simulink model "Raspberry_Audio"  (R2020a)
settings: Solver=FixedStepDiscrete  StartTime=0.0  StopTime=inf  RelTol=1e-3  EnableMultiTasking=on
InitFcn:
  | audio_equalizer_data
  | audioSignal = audioread(fullfile(matlabroot,'toolbox','signal','signal','guitartune.wav'));
  | audioSignal = int16((2^15-1)*audioSignal);
StartFcn:
  | audio_equalizer_gui
undefined symbols (not defined in the file): CoeffsMatrix1, CoeffsMatrix2, CoeffsMatrix3, dfilt
libraries: dsparch4 x3, embdlinuxlib x1, dspsrcs4 x1
CloseFcn:
  | % Delete parameters
  | clear CoeffsMatrix1 CoeffsMatrix2  CoeffsMatrix3
  | clear coeffsMatrix1   coeffsMatrix2   coeffsMatrix3
  | clear in out
  | clear audiosamplingrate
  | 
  | % Delete GUI
  | delete(findall(0, 'type', 'figure', 'Name', 'Three Band Equalizer'));
  | 
  | % Clear audio signal
  | clear audioSignal
settings Model: SimulationMode=external  ExtModeTrigDuration=100  Creator=The MathWorks, Inc.  LastModifiedBy=miche
settings SolverCC: PositivePriorityOrder=on
settings DataIOCC: LimitDataPoints=on  SaveFormat=Array  ReturnWorkspaceOutputs=off
settings OptimizationCC: ExpressionDepthLimit=2147483647  LifeSpan=Inf  MaxStackSize=64
settings DebuggingCC: UnderspecifiedInitializationDetection=Classic  MergeDetectMultiDrivingBlocksExec=none  IntegerOverflowMsg=none  ParameterOverflowMsg=none  ParameterPrecisionLossMsg=none  FcnCallInpInsideContextMsg=warning  AllowSymbolicDim=off  StateNameClashWarn=warning  SFUnexpectedBacktrackingDiag=warning  SFNoUnconditionalDefaultTransitionDiag=warning  SFExecutionAtInitializationDiag=none  IntegerSaturationMsg=none  ArithmeticOperatorsInVariantConditions=warning
settings HardwareCC: ProdBitPerPointer=32  ProdBitPerSizeT=32  ProdBitPerPtrDiffT=32  ProdLargestAtomicInteger=Long  ProdLargestAtomicFloat=Double  ProdWordSize=32  ProdHWDeviceType=ARM Compatible->ARM Cortex  UseEmbeddedCoderFeatures=off  UseSimulinkCoderFeatures=off
settings ModelReferenceCC: PropagateSignalLabelsOutOfModel=off
settings SFSimCC: SimUseLocalCustomCode=off  CustomCodeUndefinedFunction=UseInterfaceOnly
settings RTWCC: SystemTargetFile=ert.tlc  HardwareBoard=Raspberry Pi  TLCOptions=-aInlineSetEventsForThisBaseRateFcn=TLC_FALSE -aSuppressMultiTaskScheduler=TLC_FALSE -aRateBasedStepFcn=0  TemplateMakefile=ert_default_tmf  GenerateReport=on  RTWVerbose=off  RTWUseLocalCustomCode=off  Toolchain=GNU GCC Raspberry Pi  LaunchReport=on
settings CodeAppCC: ForceParamTrailComments=on  OperatorAnnotations=on  StateflowObjectComments=on  MATLABSourceComments=on
settings ERTTargetCC: MultiwordLength=2048  ERTCustomFileBanners=off  SupportContinuousTime=on  SupportNonInlinedSFcns=on  RemoveResetFunc=off  ModelStepFunctionPrototypeControlCompliant=off
settings ConfigComp: CovMetricSettings=dw  CovHtmlReporting=on  CovSaveCumulativeToWorkspaceVar=on  CovSaveSingleToWorkspaceVar=on  CovShowResultsExplorer=off  CovExternalEMLEnable=off

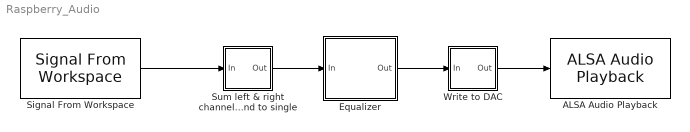
== system Raspberry_Audio ==
  ALSA Audio Playback : embdlinuxlib/ALSA Audio Playback  deviceStr='default'  sampleRateEnum=44100  queueDuration=0.5  blockPlatform=Raspberry Pi
      settings: SourceProductBaseCode=SC_BEAGLEBONE_BLUE,RASPPI
  Equalizer : Subsystem  TreatAsAtomicUnit=on
  Signal From Workspace : dspsrcs4/Signal From Workspace  X=audioSignal  Ts=1/44100  nsamps=4410  OutputAfterFinalValue=Cyclic repetition  ignoreOrWarnInputAndFrameLengths=off  OutputFrames=on
  Sum left & right channels and to single : Subsystem
  Write to DAC : Subsystem
  wires:
  Equalizer/1(Out) -> Write to DAC/1(In)
  Signal From Workspace/1 -> Sum left & right channels and to single/1(In)
  Sum left & right channels and to single/1(Out) -> Equalizer/1(In)
  Write to DAC/1(Out) -> ALSA Audio Playback/1

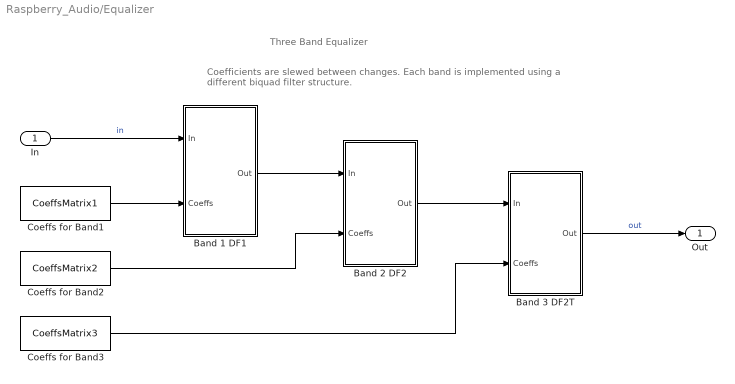
== system Raspberry_Audio/Equalizer ==
  note: Three Band Equalizer
  note: Coefficients are slewed between changes.
      | Each band is implemented using a different biquad filter structure.
  In : Inport
  Band 1 DF1 : Subsystem  TreatAsAtomicUnit=on
      settings: RTWSystemCode=Nonreusable function
  Band 2 DF2 : Subsystem  TreatAsAtomicUnit=on
      settings: RTWSystemCode=Nonreusable function
  Band 3 DF2T : Subsystem  TreatAsAtomicUnit=on
      settings: RTWSystemCode=Nonreusable function
  Coeffs for Band1 : Constant  Value=CoeffsMatrix1  VectorParams1D=off  OutDataTypeStr=single
  Coeffs for Band2 : Constant  Value=CoeffsMatrix2  VectorParams1D=off  OutDataTypeStr=single
  Coeffs for Band3 : Constant  Value=CoeffsMatrix3  VectorParams1D=off  OutDataTypeStr=single
  Out : Outport
  wires:
  In/1 -> Band 1 DF1/1(In)  "in"
  Coeffs for Band1/1 -> Band 1 DF1/2(Coeffs)
  Band 1 DF1/1(Out) -> Band 2 DF2/1(In)
  Band 2 DF2/1(Out) -> Band 3 DF2T/1(In)
  Band 3 DF2T/1(Out) -> Out/1  "out"
  Coeffs for Band2/1 -> Band 2 DF2/2(Coeffs)
  Coeffs for Band3/1 -> Band 3 DF2T/2(Coeffs)

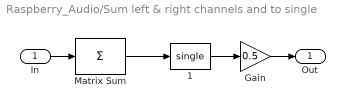
== system Raspberry_Audio/Sum left & right channels and to single ==
  In : Inport
  " 1" : DataTypeConversion  OutDataTypeStr=single
  Gain : Gain  Gain=0.5
  Matrix Sum : Sum  Inputs=+  CollapseMode=Specified dimension  CollapseDim=2
  Out : Outport
  wires:
  Gain/1 -> Out/1
  In/1 -> Matrix Sum/1
  " 1"/1 -> Gain/1
  Matrix Sum/1 -> " 1"/1

== system Raspberry_Audio/Write to DAC ==
  In : Inport
  " 5" : DataTypeConversion
  Matrix Concatenate : Concatenate  Mode=Multidimensional array  ConcatenateDimension=2
  Out : Outport
  wires:
  In/1 -> Matrix Concatenate/2, Matrix Concatenate/1
  Matrix Concatenate/1 -> " 5"/1
  " 5"/1 -> Out/1

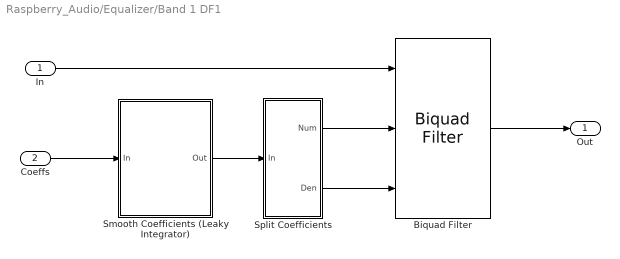
== system Raspberry_Audio/Equalizer/Band 1 DF1 ==
  In : Inport
  Coeffs : Inport  Port=2
  Biquad Filter : dsparch4/Biquad Filter  IIRFiltStruct=Direct form I  CoeffSource=Specify via dialog  BiQuadCoeffs=[1 0.3 0.4 1 0.1 0.2]  a0Flag=Warning  IC=0  ICnum=0  ICden=0  InputProcessing=Columns as channels (frame based)  denAccumFracLength=30  denProdOutputFracLength=30  secondMemoryFracLength=15  roundingMode=Floor  overflowMode=off  ScaleValues=1  optimizeScaleValues=on  ScaleValueMode=Assume all are unity and optimize  scaleValueFracLength=14  FilterSource=Input port(s)  FilterObject=dfilt.df2tsos([1 0.3 0.4],[1 0.1 0.2])
      settings: AttributesFormatString=--------------------------------------\n%<IIRFiltStruct>
  Smooth Coefficients (Leaky Integrator) : Subsystem  RTWFcnName=LeakyIntegrator  mask{b0=0.2, init_state=CoeffsMatrix1}
      mask prompts: b0 "Smoothing Coefficient: B0"; init_state "Initial State"
  Split Coefficients : Subsystem
  Out : Outport
  wires:
  Smooth Coefficients (Leaky Integrator)/1(Out) -> Split Coefficients/1(In)
  Biquad Filter/1 -> Out/1
  Coeffs/1 -> Smooth Coefficients (Leaky Integrator)/1(In)
  Split Coefficients/1(Num) -> Biquad Filter/2
  Split Coefficients/2(Den) -> Biquad Filter/3
  In/1 -> Biquad Filter/1

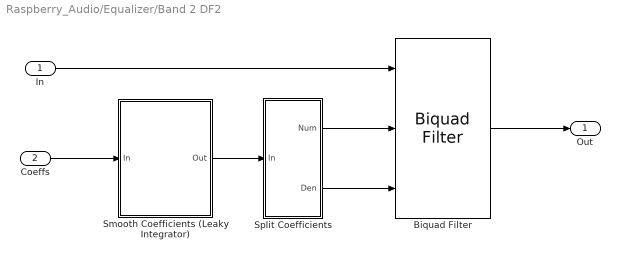
== system Raspberry_Audio/Equalizer/Band 2 DF2 ==
  In : Inport
  Coeffs : Inport  Port=2
  Biquad Filter : dsparch4/Biquad Filter  IIRFiltStruct=Direct form II  CoeffSource=Specify via dialog  BiQuadCoeffs=[1 0.3 0.4 1 0.1 0.2]  a0Flag=Warning  IC=0  ICnum=0  ICden=0  InputProcessing=Columns as channels (frame based)  denAccumFracLength=30  denProdOutputFracLength=30  secondMemoryFracLength=15  roundingMode=Floor  overflowMode=off  ScaleValues=1  optimizeScaleValues=on  ScaleValueMode=Assume all are unity and optimize  scaleValueFracLength=14  FilterSource=Input port(s)  FilterObject=dfilt.df2tsos([1 0.3 0.4],[1 0.1 0.2])
      settings: AttributesFormatString=--------------------------------------\n%<IIRFiltStruct>
  Smooth Coefficients (Leaky Integrator) : Subsystem  RTWFcnName=LeakyIntegrator  mask{b0=0.2, init_state=CoeffsMatrix2}
      mask prompts: b0 "Smoothing Coefficient: B0"; init_state "Initial State"
  Split Coefficients : Subsystem
  Out : Outport
  wires:
  Smooth Coefficients (Leaky Integrator)/1(Out) -> Split Coefficients/1(In)
  Biquad Filter/1 -> Out/1
  Coeffs/1 -> Smooth Coefficients (Leaky Integrator)/1(In)
  Split Coefficients/1(Num) -> Biquad Filter/2
  Split Coefficients/2(Den) -> Biquad Filter/3
  In/1 -> Biquad Filter/1

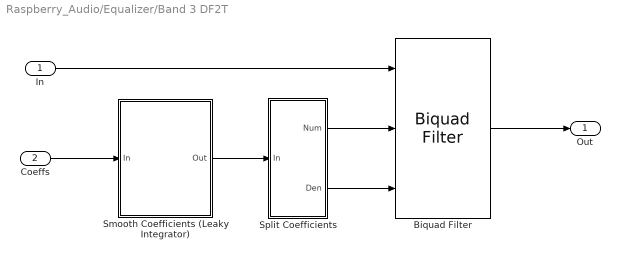
== system Raspberry_Audio/Equalizer/Band 3 DF2T ==
  In : Inport
  Coeffs : Inport  Port=2
  Biquad Filter : dsparch4/Biquad Filter  IIRFiltStruct=Direct form II transposed  CoeffSource=Specify via dialog  BiQuadCoeffs=[1 0.3 0.4 1 0.1 0.2]  a0Flag=Warning  IC=0  ICnum=0  ICden=0  InputProcessing=Columns as channels (frame based)  denAccumFracLength=30  denProdOutputFracLength=30  secondMemoryFracLength=15  roundingMode=Floor  overflowMode=off  ScaleValues=1  optimizeScaleValues=on  ScaleValueMode=Assume all are unity and optimize  scaleValueFracLength=14  FilterSource=Input port(s)  FilterObject=dfilt.df2tsos([1 0.3 0.4],[1 0.1 0.2])
      settings: AttributesFormatString=--------------------------------------\n%<IIRFiltStruct>
  Smooth Coefficients (Leaky Integrator) : Subsystem  RTWFcnName=LeakyIntegrator  mask{b0=0.2, init_state=CoeffsMatrix3}
      mask prompts: b0 "Smoothing Coefficient: B0"; init_state "Initial State"
  Split Coefficients : Subsystem
  Out : Outport
  wires:
  Smooth Coefficients (Leaky Integrator)/1(Out) -> Split Coefficients/1(In)
  Biquad Filter/1 -> Out/1
  Coeffs/1 -> Smooth Coefficients (Leaky Integrator)/1(In)
  Split Coefficients/1(Num) -> Biquad Filter/2
  Split Coefficients/2(Den) -> Biquad Filter/3
  In/1 -> Biquad Filter/1

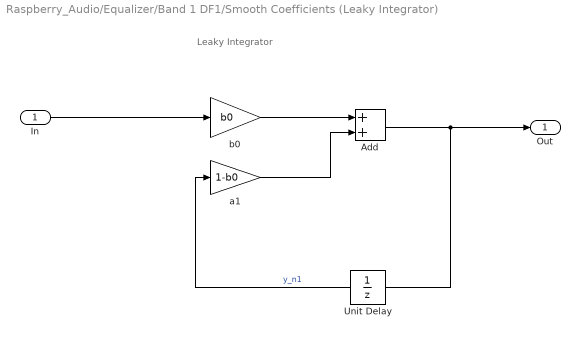
== system Raspberry_Audio/Equalizer/Band 1 DF1/Smooth Coefficients (Leaky Integrator) ==
  note: Leaky Integrator
  In : Inport
  Add : Sum  OutDataTypeStr=Inherit: Inherit via back propagation
  Unit Delay : UnitDelay  InitialCondition=init_state  SampleTime=-1  HasFrameUpgradeWarning=on
  a1 : Gain  Gain=1-b0  OutDataTypeStr=Inherit: Same as input  ParamDataTypeStr=Inherit: Same as input
  b0 : Gain  Gain=b0  OutDataTypeStr=Inherit: Same as input  ParamDataTypeStr=Inherit: Same as input
  Out : Outport
  wires:
  In/1 -> b0/1
  b0/1 -> Add/1
  Add/1 -> Out/1, Unit Delay/1
  a1/1 -> Add/2
  Unit Delay/1 -> a1/1  "y_n1"

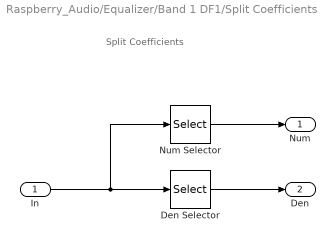
== system Raspberry_Audio/Equalizer/Band 1 DF1/Split Coefficients ==
  note: Split Coefficients
  In : Inport
  Den Selector : Selector  InputPortWidth=5  IndexOptions=Index vector (dialog)  Indices=[4 5]  OutputSizes=1
  Num Selector : Selector  InputPortWidth=5  IndexOptions=Index vector (dialog)  Indices=[1 2 3]  OutputSizes=1
  Num : Outport
  Den : Outport  Port=2
  wires:
  In/1 -> Num Selector/1, Den Selector/1
  Num Selector/1 -> Num/1
  Den Selector/1 -> Den/1

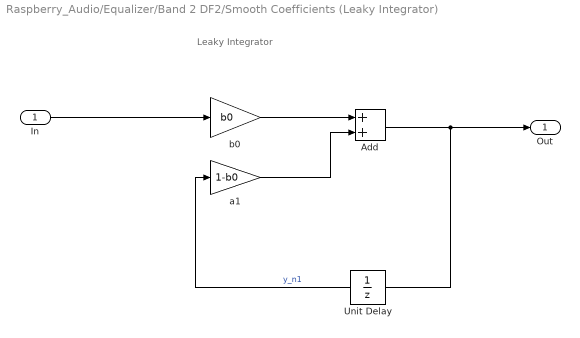
== system Raspberry_Audio/Equalizer/Band 2 DF2/Smooth Coefficients (Leaky Integrator) ==
  note: Leaky Integrator
  In : Inport
  Add : Sum  OutDataTypeStr=Inherit: Inherit via back propagation
  Unit Delay : UnitDelay  InitialCondition=init_state  SampleTime=-1  HasFrameUpgradeWarning=on
  a1 : Gain  Gain=1-b0  OutDataTypeStr=Inherit: Same as input  ParamDataTypeStr=Inherit: Same as input
  b0 : Gain  Gain=b0  OutDataTypeStr=Inherit: Same as input  ParamDataTypeStr=Inherit: Same as input
  Out : Outport
  wires:
  In/1 -> b0/1
  b0/1 -> Add/1
  Add/1 -> Out/1, Unit Delay/1
  a1/1 -> Add/2
  Unit Delay/1 -> a1/1  "y_n1"

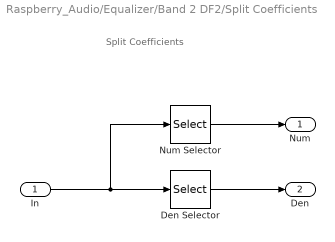
== system Raspberry_Audio/Equalizer/Band 2 DF2/Split Coefficients ==
  note: Split Coefficients
  In : Inport
  Den Selector : Selector  InputPortWidth=5  IndexOptions=Index vector (dialog)  Indices=[4 5]  OutputSizes=1
  Num Selector : Selector  InputPortWidth=5  IndexOptions=Index vector (dialog)  Indices=[1 2 3]  OutputSizes=1
  Num : Outport
  Den : Outport  Port=2
  wires:
  In/1 -> Num Selector/1, Den Selector/1
  Num Selector/1 -> Num/1
  Den Selector/1 -> Den/1

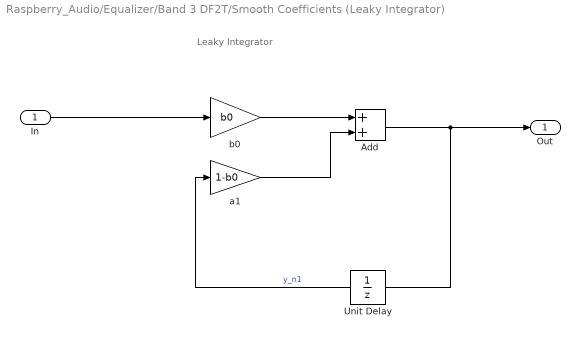
== system Raspberry_Audio/Equalizer/Band 3 DF2T/Smooth Coefficients (Leaky Integrator) ==
  note: Leaky Integrator
  In : Inport
  Add : Sum  OutDataTypeStr=Inherit: Inherit via back propagation
  Unit Delay : UnitDelay  InitialCondition=init_state  SampleTime=-1  HasFrameUpgradeWarning=on
  a1 : Gain  Gain=1-b0  OutDataTypeStr=Inherit: Same as input  ParamDataTypeStr=Inherit: Same as input
  b0 : Gain  Gain=b0  OutDataTypeStr=Inherit: Same as input  ParamDataTypeStr=Inherit: Same as input
  Out : Outport
  wires:
  In/1 -> b0/1
  b0/1 -> Add/1
  Add/1 -> Out/1, Unit Delay/1
  a1/1 -> Add/2
  Unit Delay/1 -> a1/1  "y_n1"

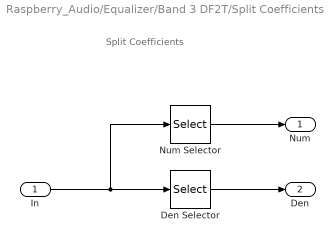
== system Raspberry_Audio/Equalizer/Band 3 DF2T/Split Coefficients ==
  note: Split Coefficients
  In : Inport
  Den Selector : Selector  InputPortWidth=5  IndexOptions=Index vector (dialog)  Indices=[4 5]  OutputSizes=1
  Num Selector : Selector  InputPortWidth=5  IndexOptions=Index vector (dialog)  Indices=[1 2 3]  OutputSizes=1
  Num : Outport
  Den : Outport  Port=2
  wires:
  In/1 -> Num Selector/1, Den Selector/1
  Num Selector/1 -> Num/1
  Den Selector/1 -> Den/1
